simulink model "CompleteHeartSim_EhsanZolfaghari"  (R2018a)
settings: Solver=ode23  StartTime=0.0  StopTime=63  RelTol=1e-3
libraries: fl_lib x41, nesl_utility x14, elec_lib x2
settings Model: Creator=RSKALA  LastModifiedBy=RSKALA
settings SolverCC: ZeroCrossAlgorithm=Adaptive
settings DebuggingCC: MaxConsecutiveZCsMsg=none

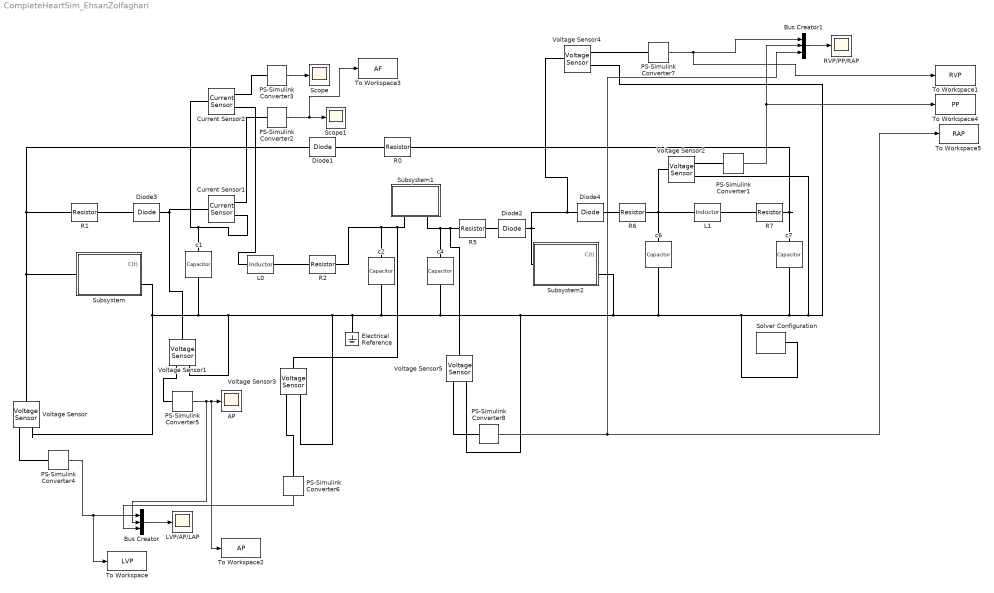
== system CompleteHeartSim_EhsanZolfaghari ==
  "AP " : Scope
  Bus Creator : BusCreator  Inputs=3
  Bus Creator1 : BusCreator  Inputs=3
  Current Sensor1 : fl_lib/Electrical/Electrical Sensors/Current Sensor
  Current Sensor2 : fl_lib/Electrical/Electrical Sensors/Current Sensor
  Diode1 : fl_lib/Electrical/Electrical Elements/Diode  Vf=0.001 V  Ron=0.003 Ohm  Goff=1e-8 1/Ohm  i_specify=off  i_priority=None  i=0 A  i_nominal_specify=off  i_nominal_unit=A  i_nominal_value=1  v_specify=off  v_priority=None  v=0 V  v_nominal_specify=off  v_nominal_unit=V  v_nominal_value=1
  Diode2 : fl_lib/Electrical/Electrical Elements/Diode  Vf=0.001 V  Ron=0.004 Ohm  Goff=1e-8 1/Ohm  i_specify=off  i_priority=None  i=0 A  i_nominal_specify=off  i_nominal_unit=A  i_nominal_value=1  v_specify=off  v_priority=None  v=0 V  v_nominal_specify=off  v_nominal_unit=V  v_nominal_value=1
  Diode3 : fl_lib/Electrical/Electrical Elements/Diode  Vf=0.001 V  Ron=0.003 Ohm  Goff=1e-8 1/Ohm  i_specify=off  i_priority=None  i=0 A  i_nominal_specify=off  i_nominal_unit=A  i_nominal_value=1  v_specify=off  v_priority=None  v=0 V  v_nominal_specify=off  v_nominal_unit=V  v_nominal_value=1
  Diode4 : fl_lib/Electrical/Electrical Elements/Diode  Vf=0.001 V  Ron=0.004 Ohm  Goff=1e-8 1/Ohm  i_specify=off  i_priority=None  i=0 A  i_nominal_specify=off  i_nominal_unit=A  i_nominal_value=1  v_specify=off  v_priority=None  v=0 V  v_nominal_specify=off  v_nominal_unit=V  v_nominal_value=1
  Electrical Reference : fl_lib/Electrical/Electrical Elements/Electrical Reference
  L0 : elec_lib/Passive Devices/Inductor  l=0.01 H  L_tol=30  enable_L_tol=0  tol_distribution=1  nSigma=4  r=0 Ohm  g=1e-9 1/Ohm  enable_operating_limits=0  operating_limit_action=2  max_working_current=1 A  power_rating=1 W  enable_faults=0  fault_action=1  lambdaPercent=50  k_faulted=0.9999  turnsShort=0  openCct=0  groundShort=0  groundShortG=0 1/Ohm  tau_fault=1e-3 s  enable_temporal_fault=0  t_fault=1 s  enable_behavioral_fault=0  max_permissible_voltage=100 V  n_fail_on_voltage=1  max_permissible_current=1 A  t_fail_on_current=1 s  i_L_specify=off  i_L_priority=High  i_L=0 A  i_L_nominal_specify=off  i_L_nominal_unit=A  i_L_nominal_value=1
      settings: SourceProductName=Simscape Electronics  SourceProductBaseCode=SN
  L1 : elec_lib/Passive Devices/Inductor  l=0.002 H  L_tol=20  enable_L_tol=0  tol_distribution=1  nSigma=4  r=0 Ohm  g=1e-9 1/Ohm  enable_operating_limits=0  operating_limit_action=2  max_working_current=1 A  power_rating=1 W  enable_faults=0  fault_action=1  lambdaPercent=50  k_faulted=0.9999  turnsShort=0  openCct=0  groundShort=0  groundShortG=0 1/Ohm  tau_fault=1e-3 s  enable_temporal_fault=0  t_fault=1 s  enable_behavioral_fault=0  max_permissible_voltage=100 V  n_fail_on_voltage=1  max_permissible_current=1 A  t_fail_on_current=1 s  i_L_specify=off  i_L_priority=High  i_L=0 A  i_L_nominal_specify=off  i_L_nominal_unit=A  i_L_nominal_value=1
      settings: SourceProductName=Simscape Electronics  SourceProductBaseCode=SN
  "LVP/AP/LAP " : Scope
  PS-Simulink Converter{1..8} (8 alike) : nesl_utility/PS-Simulink Converter  PhysicalDomain=network_engine_domain  SubClassName=ps_output  LeftPortType=input  RightPortType=output  PseudoPeriodic=off  Frequencies=[]  Unit=1  AffineConversion=on
  R0 : fl_lib/Electrical/Electrical Elements/Resistor  R=0.004 Ohm  i_specify=off  i_priority=None  i=0 A  i_nominal_specify=off  i_nominal_unit=A  i_nominal_value=1  v_specify=off  v_priority=None  v=0 V  v_nominal_specify=off  v_nominal_unit=V  v_nominal_value=1
  R1 : fl_lib/Electrical/Electrical Elements/Resistor  R=0.004 Ohm  i_specify=off  i_priority=None  i=0 A  i_nominal_specify=off  i_nominal_unit=A  i_nominal_value=1  v_specify=off  v_priority=None  v=0 V  v_nominal_specify=off  v_nominal_unit=V  v_nominal_value=1
  R2 : fl_lib/Electrical/Electrical Elements/Resistor  R=0.52 Ohm  i_specify=off  i_priority=None  i=0 A  i_nominal_specify=off  i_nominal_unit=A  i_nominal_value=1  v_specify=off  v_priority=None  v=0 V  v_nominal_specify=off  v_nominal_unit=V  v_nominal_value=1
  R5 : fl_lib/Electrical/Electrical Elements/Resistor  R=0.004 Ohm  i_specify=off  i_priority=None  i=0 A  i_nominal_specify=off  i_nominal_unit=A  i_nominal_value=1  v_specify=off  v_priority=None  v=0 V  v_nominal_specify=off  v_nominal_unit=V  v_nominal_value=1
  R6 : fl_lib/Electrical/Electrical Elements/Resistor  R=0.002 Ohm  i_specify=off  i_priority=None  i=0 A  i_nominal_specify=off  i_nominal_unit=A  i_nominal_value=1  v_specify=off  v_priority=None  v=0 V  v_nominal_specify=off  v_nominal_unit=V  v_nominal_value=1
  R7 : fl_lib/Electrical/Electrical Elements/Resistor  R=0.2 Ohm  i_specify=off  i_priority=None  i=0 A  i_nominal_specify=off  i_nominal_unit=A  i_nominal_value=1  v_specify=off  v_priority=None  v=0 V  v_nominal_specify=off  v_nominal_unit=V  v_nominal_value=1
  RVP/PP/RAP : Scope
  Scope : Scope
  Scope1 : Scope
  Solver Configuration : nesl_utility/Solver Configuration  PhysicalDomain=network_engine_domain  SubClassName=solver  LeftPortType=input  RightPortType=generic  Tones=[]  Harmonics=[]  SimulateNoise=off  Profile=off  UseLocalSampling=off  EnableSwitchedLinearOptims=on  FrequencyDomain=off  UseCCode=off  RelTol=0.001  AbsTol=1e-06  MinStep=1e-09  ToWorkspace=off  RevertToSquareIcSolve=off  NumHomotopyIterations=100  PhasorMode=off  PhasorModeNumHarmonics=1  DoDC=off  ResidualTolerance=1e-09  UseLocalSolver=off  LocalSolverChoice=NE_BACKWARD_EULER_ADVANCER  LocalSolverSampleTime=0.001  DoFixedCost=off  MaxNonlinIter=3  MaxModeIter=2  LinearAlgebra=Sparse  EquationFormulation=NE_TIME_EF  DelaysMemoryBudget=1024  AutomaticFiltering=on  FilteringTimeConstant=0.001
  Subsystem : Subsystem
  Subsystem1 : Subsystem
  Subsystem2 : Subsystem
  To Workspace : ToWorkspace  VariableName=LVP  SaveFormat=Timeseries  SampleTime=-1
  To Workspace1 : ToWorkspace  VariableName=RVP  SaveFormat=Timeseries  SampleTime=-1
  To Workspace2 : ToWorkspace  VariableName=AP  SaveFormat=Timeseries  SampleTime=-1
  To Workspace3 : ToWorkspace  VariableName=AF  SaveFormat=Timeseries  SampleTime=-1
  To Workspace4 : ToWorkspace  VariableName=PP  SaveFormat=Timeseries  SampleTime=-1
  To Workspace5 : ToWorkspace  VariableName=RAP  SaveFormat=Timeseries  SampleTime=-1
  Voltage Sensor{,1..5} (6 alike) : fl_lib/Electrical/Electrical Sensors/Voltage Sensor
  c1 : fl_lib/Electrical/Electrical Elements/Capacitor  c=0.75 F  r=1e-6 Ohm  g=0 1/Ohm  i_specify=off  i_priority=None  i=0 A  i_nominal_specify=off  i_nominal_unit=A  i_nominal_value=1  v_specify=off  v_priority=None  v=0 V  v_nominal_specify=off  v_nominal_unit=V  v_nominal_value=1  vc_specify=off  vc_priority=High  vc=0 V  vc_nominal_specify=off  vc_nominal_unit=V  vc_nominal_value=1
  c2 : fl_lib/Electrical/Electrical Elements/Capacitor  c=1 F  r=1e-6 Ohm  g=0 1/Ohm  i_specify=off  i_priority=None  i=0 A  i_nominal_specify=off  i_nominal_unit=A  i_nominal_value=1  v_specify=off  v_priority=None  v=0 V  v_nominal_specify=off  v_nominal_unit=V  v_nominal_value=1  vc_specify=off  vc_priority=High  vc=0 V  vc_nominal_specify=off  vc_nominal_unit=V  vc_nominal_value=1
  c4 : fl_lib/Electrical/Electrical Elements/Capacitor  c=10 F  r=1e-6 Ohm  g=0 1/Ohm  i_specify=off  i_priority=None  i=0 A  i_nominal_specify=off  i_nominal_unit=A  i_nominal_value=1  v_specify=off  v_priority=None  v=0 V  v_nominal_specify=off  v_nominal_unit=V  v_nominal_value=1  vc_specify=off  vc_priority=High  vc=0 V  vc_nominal_specify=off  vc_nominal_unit=V  vc_nominal_value=1
  c6 : fl_lib/Electrical/Electrical Elements/Capacitor  c=1.5 F  r=1e-6 Ohm  g=0 1/Ohm  i_specify=off  i_priority=None  i=0 A  i_nominal_specify=off  i_nominal_unit=A  i_nominal_value=1  v_specify=off  v_priority=None  v=0 V  v_nominal_specify=off  v_nominal_unit=V  v_nominal_value=1  vc_specify=off  vc_priority=High  vc=0 V  vc_nominal_specify=off  vc_nominal_unit=V  vc_nominal_value=1
  c7 : fl_lib/Electrical/Electrical Elements/Capacitor  c=5 F  r=1e-6 Ohm  g=0 1/Ohm  i_specify=off  i_priority=None  i=0 A  i_nominal_specify=off  i_nominal_unit=A  i_nominal_value=1  v_specify=off  v_priority=None  v=0 V  v_nominal_specify=off  v_nominal_unit=V  v_nominal_value=1  vc_specify=off  vc_priority=High  vc=0 V  vc_nominal_specify=off  vc_nominal_unit=V  vc_nominal_value=1
  wires:
  PS-Simulink Converter2/1 -> To Workspace3/1, Scope1/1
  PS-Simulink Converter3/1 -> Scope/1
  PS-Simulink Converter5/1 -> Bus Creator/2, To Workspace2/1, "AP "/1
  PS-Simulink Converter6/1 -> Bus Creator/3
  PS-Simulink Converter7/1 -> To Workspace1/1, Bus Creator1/1
  Bus Creator/1 -> "LVP/AP/LAP "/1
  PS-Simulink Converter8/1 -> Bus Creator1/3, To Workspace5/1
  Bus Creator1/1 -> RVP/PP/RAP/1
  PS-Simulink Converter4/1 -> To Workspace/1, Bus Creator/1
  PS-Simulink Converter1/1 -> Bus Creator1/2, To Workspace4/1
  connections:
  Subsystem/LConn1 -- R1/LConn1 -- Diode1/RConn1 -- Voltage Sensor/LConn1
  Diode3/RConn1 -- Current Sensor1/LConn1 -- Voltage Sensor1/LConn1
  Electrical Reference/LConn1 -- Voltage Sensor3/RConn2 -- Voltage Sensor1/RConn2 -- c1/RConn1 -- Voltage Sensor/RConn2 -- Subsystem/RConn1 -- Voltage Sensor5/RConn2 -- Voltage Sensor4/RConn2 -- Voltage Sensor2/RConn2 -- c7/RConn1 -- Solver Configuration/RConn1 -- c6/RConn1 -- Subsystem2/RConn1 -- c4/RConn1 -- c2/RConn1
  c2/LConn1 -- Voltage Sensor3/LConn1 -- Subsystem1/RConn1 -- R2/RConn1
  R1/RConn1 -- Diode3/LConn1
  L0/RConn1 -- R2/LConn1
  PS-Simulink Converter2/LConn1 -- Current Sensor1/RConn1
  c1/LConn1 -- Current Sensor1/RConn2 -- Current Sensor2/LConn1
  L0/LConn1 -- Current Sensor2/RConn2
  Diode1/LConn1 -- R0/LConn1
  R5/LConn1 -- Subsystem1/RConn2 -- c4/LConn1 -- Voltage Sensor5/LConn1
  Diode2/LConn1 -- R5/RConn1
  Diode2/RConn1 -- Voltage Sensor4/LConn1 -- Diode4/LConn1 -- Subsystem2/LConn1
  R6/LConn1 -- Diode4/RConn1
  c6/LConn1 -- Voltage Sensor2/LConn1 -- L1/LConn1 -- R6/RConn1
  R7/LConn1 -- L1/RConn1
  R7/RConn1 -- R0/RConn1 -- c7/LConn1
  Voltage Sensor2/RConn1 -- PS-Simulink Converter1/LConn1
  Current Sensor2/RConn1 -- PS-Simulink Converter3/LConn1
  PS-Simulink Converter4/LConn1 -- Voltage Sensor/RConn1
  Voltage Sensor1/RConn1 -- PS-Simulink Converter5/LConn1
  Voltage Sensor3/RConn1 -- PS-Simulink Converter6/LConn1
  PS-Simulink Converter7/LConn1 -- Voltage Sensor4/RConn1
  PS-Simulink Converter8/LConn1 -- Voltage Sensor5/RConn1

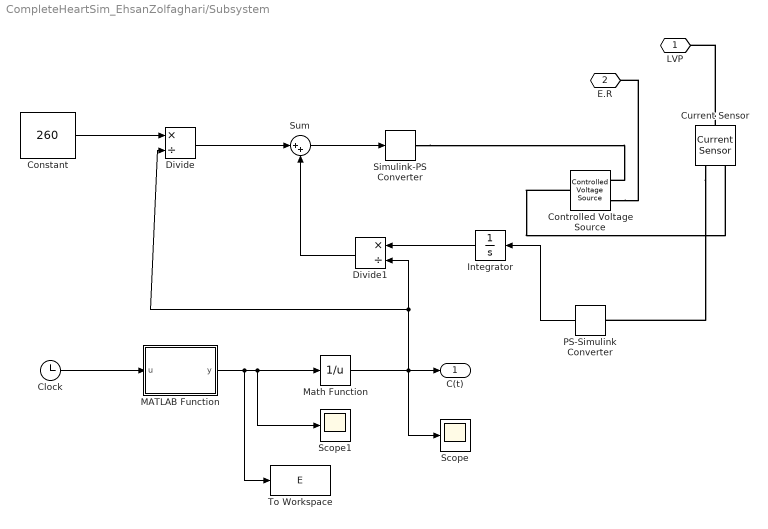
== system CompleteHeartSim_EhsanZolfaghari/Subsystem ==
  Clock : Clock
  Constant : Constant  Value=260
  Controlled Voltage Source : fl_lib/Electrical/Electrical Sources/Controlled Voltage Source
  Current Sensor : fl_lib/Electrical/Electrical Sensors/Current Sensor
  Divide : Product  Inputs=*/
  Divide1 : Product  Inputs=*/
  Integrator : Integrator
  MATLAB Function : MATLAB Function  TreatAsAtomicUnit=on
  Math Function : Math  Operator=reciprocal  RndMeth=Zero  SaturateOnIntegerOverflow=on
  PS-Simulink Converter : nesl_utility/PS-Simulink Converter  PhysicalDomain=network_engine_domain  SubClassName=ps_output  LeftPortType=input  RightPortType=output  PseudoPeriodic=off  Frequencies=[]  Unit=1  AffineConversion=off
  Scope : Scope
  Scope1 : Scope
  Simulink-PS Converter : nesl_utility/Simulink-PS Converter  PhysicalDomain=network_engine_domain  SubClassName=ps_input  LeftPortType=input  RightPortType=output  PseudoPeriodic=off  Frequencies=[]  NoiseDistribution=none  NoiseParameters=[]  Unit=1  AffineConversion=off  FilteringAndDerivatives=provide  SimscapeFilterOrder=1  InputFilterTimeConstant=0.001  UdotUserProvided=0
  Sum : Sum  Inputs=|++
  To Workspace : ToWorkspace  VariableName=E  SaveFormat=Timeseries  SampleTime=-1
  "LVP " : PMIOPort  Side=Left
  E.R : PMIOPort  Port=2  Side=Right
  "C(t) " : Outport
  wires:
  Constant/1 -> Divide/1
  Divide/1 -> Sum/1
  Sum/1 -> Simulink-PS Converter/1
  Divide1/1 -> Sum/2
  Integrator/1 -> Divide1/1
  Clock/1 -> MATLAB Function/1(u)
  MATLAB Function/1(y) -> To Workspace/1, Scope1/1, Math Function/1
  Math Function/1 -> Scope/1, Divide/2, Divide1/2, "C(t) "/1
  PS-Simulink Converter/1 -> Integrator/1
  connections:
  Simulink-PS Converter/RConn1 -- Controlled Voltage Source/RConn1
  Controlled Voltage Source/LConn1 -- Current Sensor/RConn2
  Current Sensor/RConn1 -- PS-Simulink Converter/LConn1
  Current Sensor/LConn1 -- "LVP "/RConn1
  Controlled Voltage Source/RConn2 -- E.R/RConn1

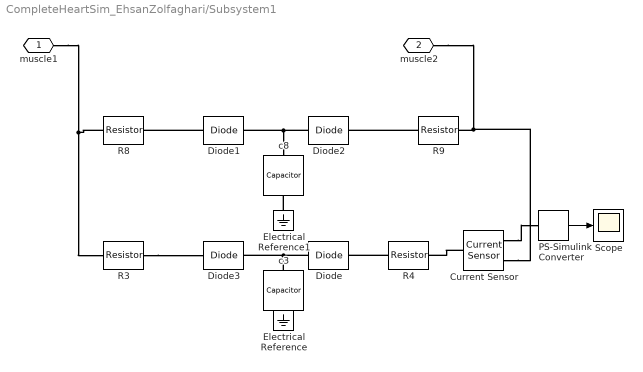
== system CompleteHeartSim_EhsanZolfaghari/Subsystem1 ==
  Current Sensor : fl_lib/Electrical/Electrical Sensors/Current Sensor
  Diode{,1..3} (4 alike) : fl_lib/Electrical/Electrical Elements/Diode  Vf=0.001 V  Ron=0.004 Ohm  Goff=1e-8 1/Ohm  i_specify=off  i_priority=None  i=0 A  i_nominal_specify=off  i_nominal_unit=A  i_nominal_value=1  v_specify=off  v_priority=None  v=0 V  v_nominal_specify=off  v_nominal_unit=V  v_nominal_value=1
  Electrical Reference : fl_lib/Electrical/Electrical Elements/Electrical Reference
  Electrical Reference1 : fl_lib/Electrical/Electrical Elements/Electrical Reference
  PS-Simulink Converter : nesl_utility/PS-Simulink Converter  PhysicalDomain=network_engine_domain  SubClassName=ps_output  LeftPortType=input  RightPortType=output  PseudoPeriodic=off  Frequencies=[]  Unit=1  AffineConversion=off
  R3 : fl_lib/Electrical/Electrical Elements/Resistor  R=8.5 Ohm  i_specify=off  i_priority=None  i=0 A  i_nominal_specify=off  i_nominal_unit=A  i_nominal_value=1  v_specify=off  v_priority=None  v=0 V  v_nominal_specify=off  v_nominal_unit=V  v_nominal_value=1
  R4 : fl_lib/Electrical/Electrical Elements/Resistor  R=0.1 Ohm  i_specify=off  i_priority=None  i=0 A  i_nominal_specify=off  i_nominal_unit=A  i_nominal_value=1  v_specify=off  v_priority=None  v=0 V  v_nominal_specify=off  v_nominal_unit=V  v_nominal_value=1
  R8 : fl_lib/Electrical/Electrical Elements/Resistor  R=0.95 Ohm  i_specify=off  i_priority=None  i=0 A  i_nominal_specify=off  i_nominal_unit=A  i_nominal_value=1  v_specify=off  v_priority=None  v=0 V  v_nominal_specify=off  v_nominal_unit=V  v_nominal_value=1
  R9 : fl_lib/Electrical/Electrical Elements/Resistor  R=0.023 Ohm  i_specify=off  i_priority=None  i=0 A  i_nominal_specify=off  i_nominal_unit=A  i_nominal_value=1  v_specify=off  v_priority=None  v=0 V  v_nominal_specify=off  v_nominal_unit=V  v_nominal_value=1
  Scope : Scope
  c3 : fl_lib/Electrical/Electrical Elements/Capacitor  c=10 F  r=1e-6 Ohm  g=0 1/Ohm  i_specify=off  i_priority=None  i=0 A  i_nominal_specify=off  i_nominal_unit=A  i_nominal_value=1  v_specify=off  v_priority=None  v=0 V  v_nominal_specify=off  v_nominal_unit=V  v_nominal_value=1  vc_specify=off  vc_priority=High  vc=0 V  vc_nominal_specify=off  vc_nominal_unit=V  vc_nominal_value=1
  c8 : fl_lib/Electrical/Electrical Elements/Capacitor  c=12.5 F  r=1e-6 Ohm  g=0 1/Ohm  i_specify=off  i_priority=None  i=0 A  i_nominal_specify=off  i_nominal_unit=A  i_nominal_value=1  v_specify=off  v_priority=None  v=0 V  v_nominal_specify=off  v_nominal_unit=V  v_nominal_value=1  vc_specify=off  vc_priority=High  vc=0 V  vc_nominal_specify=off  vc_nominal_unit=V  vc_nominal_value=1
  "muscle1 " : PMIOPort  Side=Right
  "muscle2 " : PMIOPort  Port=2  Side=Right
  wires:
  PS-Simulink Converter/1 -> Scope/1
  connections:
  "muscle2 "/RConn1 -- Current Sensor/RConn2 -- R9/RConn1
  R9/LConn1 -- Diode2/RConn1
  Diode2/LConn1 -- c8/LConn1 -- Diode1/RConn1
  Diode1/LConn1 -- R8/RConn1
  "muscle1 "/RConn1 -- R8/LConn1 -- R3/LConn1
  R3/RConn1 -- Diode3/LConn1
  Diode/LConn1 -- Diode3/RConn1 -- c3/LConn1
  R4/LConn1 -- Diode/RConn1
  Current Sensor/LConn1 -- R4/RConn1
  Current Sensor/RConn1 -- PS-Simulink Converter/LConn1
  c3/RConn1 -- Electrical Reference/LConn1
  Electrical Reference1/LConn1 -- c8/RConn1

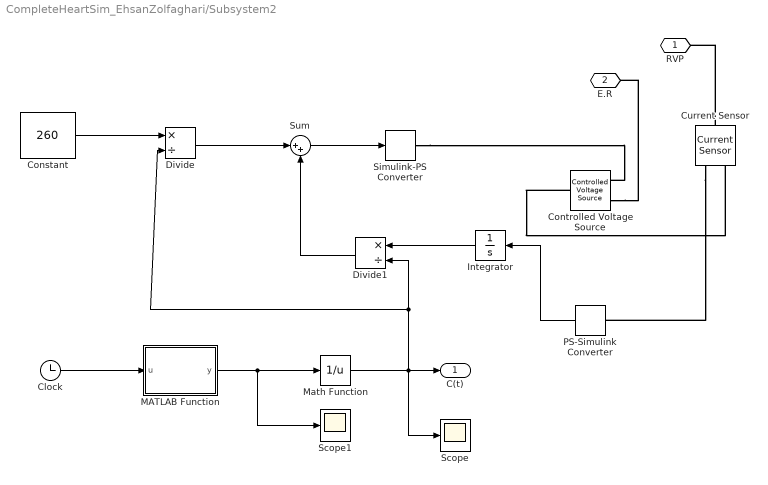
== system CompleteHeartSim_EhsanZolfaghari/Subsystem2 ==
  Clock : Clock
  Constant : Constant  Value=260
  Controlled Voltage Source : fl_lib/Electrical/Electrical Sources/Controlled Voltage Source
  Current Sensor : fl_lib/Electrical/Electrical Sensors/Current Sensor
  Divide : Product  Inputs=*/
  Divide1 : Product  Inputs=*/
  Integrator : Integrator
  MATLAB Function : MATLAB Function  TreatAsAtomicUnit=on
  Math Function : Math  Operator=reciprocal  RndMeth=Round  SaturateOnIntegerOverflow=on
  PS-Simulink Converter : nesl_utility/PS-Simulink Converter  PhysicalDomain=network_engine_domain  SubClassName=ps_output  LeftPortType=input  RightPortType=output  PseudoPeriodic=off  Frequencies=[]  Unit=1  AffineConversion=off
  Scope : Scope
  Scope1 : Scope
  Simulink-PS Converter : nesl_utility/Simulink-PS Converter  PhysicalDomain=network_engine_domain  SubClassName=ps_input  LeftPortType=input  RightPortType=output  PseudoPeriodic=off  Frequencies=[]  NoiseDistribution=none  NoiseParameters=[]  Unit=1  AffineConversion=off  FilteringAndDerivatives=provide  SimscapeFilterOrder=1  InputFilterTimeConstant=0.001  UdotUserProvided=0
  Sum : Sum  Inputs=|++
  "RVP " : PMIOPort  Side=Left
  E.R : PMIOPort  Port=2  Side=Right
  "C(t) " : Outport
  wires:
  PS-Simulink Converter/1 -> Integrator/1
  Math Function/1 -> "C(t) "/1, Divide1/2, Divide/2, Scope/1
  MATLAB Function/1(y) -> Math Function/1, Scope1/1
  Clock/1 -> MATLAB Function/1(u)
  Integrator/1 -> Divide1/1
  Divide1/1 -> Sum/2
  Sum/1 -> Simulink-PS Converter/1
  Divide/1 -> Sum/1
  Constant/1 -> Divide/1
  connections:
  Controlled Voltage Source/RConn2 -- E.R/RConn1
  Current Sensor/LConn1 -- "RVP "/RConn1
  Current Sensor/RConn1 -- PS-Simulink Converter/LConn1
  Controlled Voltage Source/LConn1 -- Current Sensor/RConn2
  Simulink-PS Converter/RConn1 -- Controlled Voltage Source/RConn1

== matlab function CompleteHeartSim_EhsanZolfaghari/Subsystem2/MATLAB Function ==
  data: u input; y output
function y = fcn(u)

Emin = 0.06;
Emax =2.7;
HR = 75;
tc=60./HR;
Tmax=0.2+0.15.*tc;
uu = u-floor(u/tc)*tc;
y = ((Emax-Emin).*(1.55.*((uu)./Tmax./0.7).^1.9./(1+((uu)...
    ./Tmax./0.7).^1.9).*(1/(1+((uu)./Tmax./1.17)^21.9)))+Emin);
end

== matlab function CompleteHeartSim_EhsanZolfaghari/Subsystem/MATLAB Function ==
  data: u input; y output
function y = fcn(u)

Emin = 0.05;
Emax = 2.7;
HR = 75;
tc=60./HR;
Tmax=0.2+0.15.*tc;
uu = u-floor(u/tc)*tc;
y = ((Emax-Emin).*(1.55.*((uu)./Tmax./0.7).^1.9./(1+((uu)...
    ./Tmax./0.7).^1.9).*(1/(1+((uu)./Tmax./1.17)^21.9)))+Emin);
end
